simulink model "Filter"  (R2020b)
settings: Solver=FixedStepAuto  StartTime=0.0  StopTime=10.0  FixedStep=0.2  RelTol=1e-3
settings Model: Creator=DELL  LastModifiedBy=DELL
settings DataIOCC: SaveOutput=off  SaveTime=off

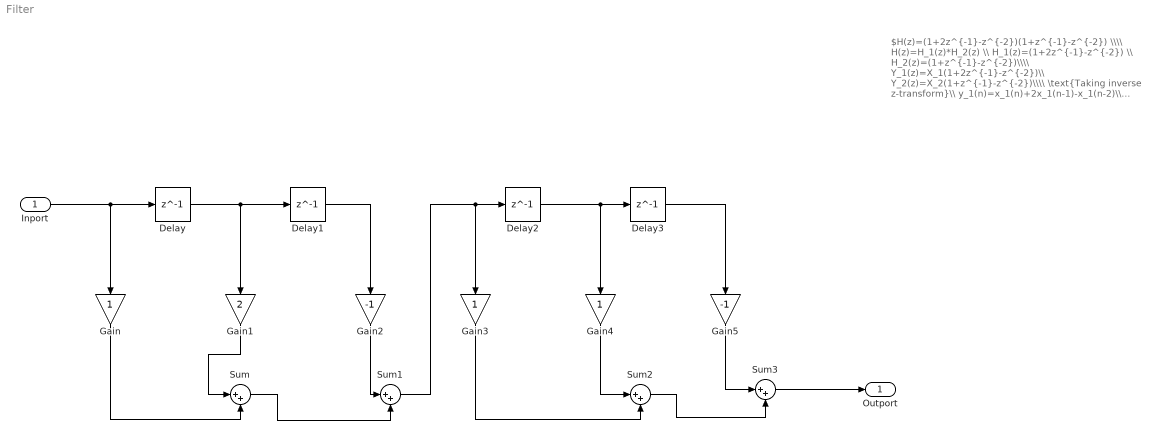
== system Filter ==
  note: $H(z)=(1+2z^{-1}-z^{-2})(1+z^{-1}-z^{-2}) \\\\ H(z)=H_1(z)*H_2(z) \\ H_1(z)=(1+2z^{-1}-z^{-2}) \\ H_2(z)=(1+z^{-1}-z^{-2})\\\\ Y_1(z)=X_1(1+2z^{-1}-z^{-2})\\ Y_2(z)=X_2(1+z^{-1}-z^{-2})\\\\ \text{Taking inverse z-transform}\\ y_1(n)=x_1(n)+2x_1(n-1)-x_1(n-2)\\ y_2(n)=x_2(n)+x_2(n-1)-x_2(n-2)$
  Inport : Inport  OutDataTypeStr=double  PortDimensions=1  SampleTime=[0.20000000000000001,0]
  Delay{,1..3} (4 alike) : Delay  DelayLength=1
  Gain : Gain
  Gain1 : Gain  Gain=2
  Gain2 : Gain  Gain=-1
  Gain3 : Gain
  Gain4 : Gain
  Gain5 : Gain  Gain=-1
  Sum{,1..3} (4 alike) : Sum  Inputs=|++
  Outport : Outport  OutDataTypeStr=double  PortDimensions=1  SampleTime=[0.20000000000000001,0]
  wires:
  Delay/1 -> Delay1/1, Gain1/1
  Inport/1 -> Delay/1, Gain/1
  Gain4/1 -> Sum2/1
  Delay3/1 -> Gain5/1
  Sum1/1 -> Delay2/1, Gain3/1
  Sum2/1 -> Sum3/2
  Gain3/1 -> Sum2/2
  Delay2/1 -> Delay3/1, Gain4/1
  Gain2/1 -> Sum1/1
  Sum/1 -> Sum1/2
  Gain1/1 -> Sum/1
  Gain5/1 -> Sum3/1
  Gain/1 -> Sum/2
  Sum3/1 -> Outport/1
  Delay1/1 -> Gain2/1
